simulink model "mras_absolute_error"  (R2019b)
settings: Solver=VariableStepAuto  StartTime=0.0  StopTime=50  RelTol=1e-3
values from neighbouring files (symbols this model uses):
  Am = [1 7 12]    [Second_order_system.m]
  b = 7    [Second_order_system.m]
  Bm = 12    [Second_order_system.m]
  gamma = 1.2    [Second_order_system.m]
settings Model: Creator=Mustafa Sezer  LastModifiedBy=Mustafa Sezer

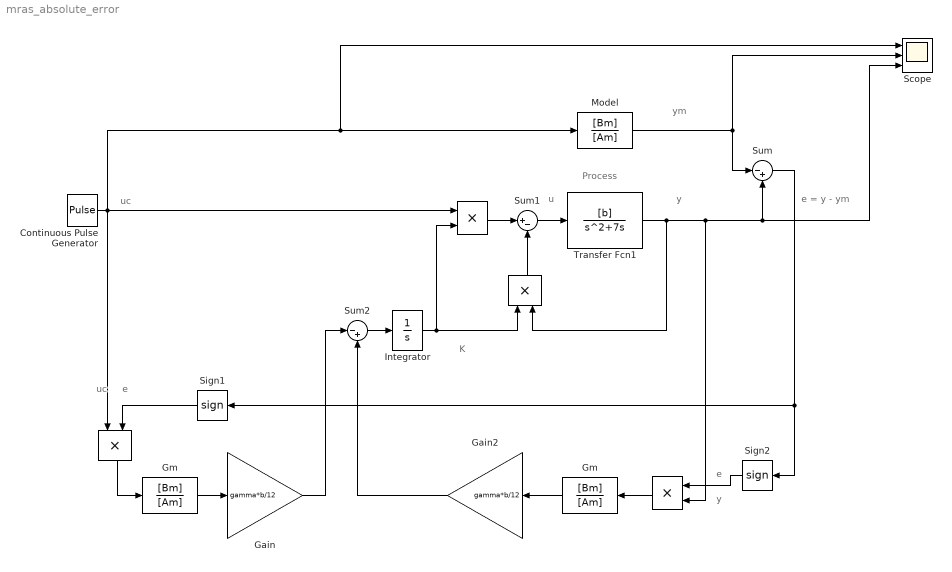
== system mras_absolute_error ==
  note: y
  note: uc
  note: K
  note: e = y - ym
  note: e
  note: Process
  note: y
  note: ym
  note: e
  note: u
  note: uc
  " " : Product
  " " : Product
  " " : Product
  "     " : Product
  Continuous Pulse Generator : DiscretePulseGenerator  PulseType=Time based  Period=20  PulseWidth=50
  Gain : Gain  Gain=gamma*b/12
  Gain2 : Gain  Gain=gamma*b/12
  "Gm " : TransferFcn  Numerator=[Bm]  Denominator=[Am]
  "Gm  " : TransferFcn  Numerator=[Bm]  Denominator=[Am]
  Integrator : Integrator
  Model : TransferFcn  Numerator=[Bm]  Denominator=[Am]
  Scope : Scope  NumInputPorts=3
  Sign1 : Signum
  Sign2 : Signum
  Sum : Sum  Inputs=|-+
  Sum1 : Sum  Inputs=|+-
  Sum2 : Sum  Inputs=|-+
  Transfer Fcn1 : TransferFcn  Numerator=[b]  Denominator=[1 7 0]
  wires:
  "Gm "/1 -> Gain2/1
  Integrator/1 -> " "/1, "     "/2
  Sum1/1 -> Transfer Fcn1/1
  Continuous Pulse Generator/1 -> "     "/1, Scope/1, Model/1, " "/1
  "     "/1 -> Sum1/1
  Sum/1 -> Sign2/1, Sign1/1
  " "/1 -> "Gm  "/1
  Transfer Fcn1/1 -> " "/2, Sum/2, Scope/3, " "/2
  Gain/1 -> Sum2/1
  Model/1 -> Sum/1, Scope/2
  "Gm  "/1 -> Gain/1
  " "/1 -> Sum1/2
  Gain2/1 -> Sum2/2
  Sum2/1 -> Integrator/1
  " "/1 -> "Gm "/1
  Sign2/1 -> " "/1
  Sign1/1 -> " "/2
